simulink model "Boost_Converter"  (R2022b)
settings: Solver=VariableStepAuto  StartTime=0.0  StopTime=0.1  RelTol=1e-3
libraries: spsSeriesRLCBranchLib x3, spsMultimeterLib x2, spsDiodeLib x1, spsMeanLib x1, spsMosfetLib x1, spsPWMGeneratorDCDCLib x1, spsDCVoltageSourceLib x1, sps_lib x1
settings Model: Creator=Biplov Jha  LastModifiedBy=Biplov Jha

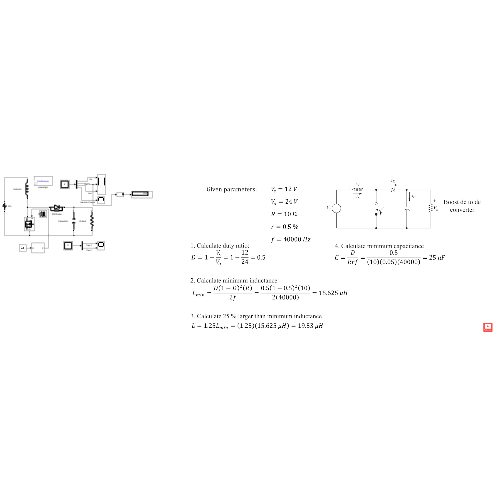
[thumbnail: Simulink's stored preview of the top-level diagram]
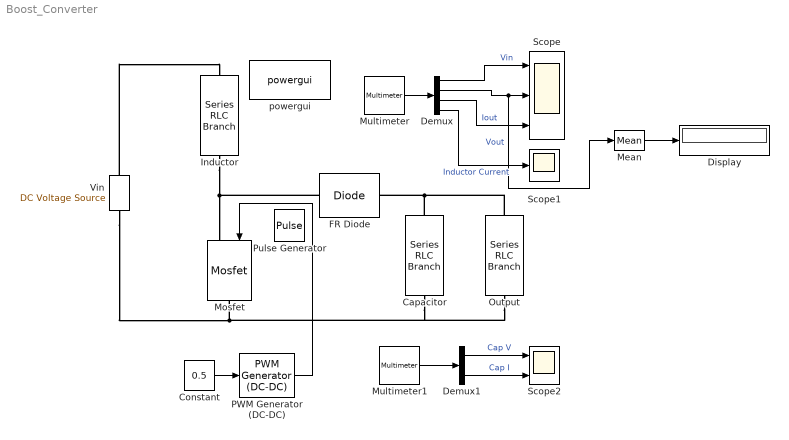
== system Boost_Converter ==
  Capacitor : spsSeriesRLCBranchLib/Series RLC Branch  LConnTagsString=__new0  RConnTagsString=__new0  BranchType=C  Resistance=1  Inductance=1e-3  SetiL0=off  InitialCurrent=0  Capacitance=25e-6  Setx0=off  InitialVoltage=0  Measurements=Branch voltage and current
  Constant : Constant  Value=0.5
  Demux : Demux
  Demux1 : Demux  Outputs=2
  Display : Display
  FR Diode : spsDiodeLib/Diode  Ron=0.001  Lon=0  Vf=0.8  IC=0  UseSnubber=0  Rs=500  Cs=250e-9  Measurements=off
  Inductor : spsSeriesRLCBranchLib/Series RLC Branch  LConnTagsString=__new0  RConnTagsString=__new0  BranchType=L  Resistance=1  Inductance=20e-6  SetiL0=off  InitialCurrent=0  Capacitance=1e-6  Setx0=off  InitialVoltage=0  Measurements=Branch current
  Mean : spsMeanLib/Mean  Freq=60  Vinit=0  Ts=0
  Mosfet : spsMosfetLib/Mosfet  Ron=0.1  Lon=0  Rd=0.01  Vfd=0  IC=0  Rs=1e5  Cs=inf  Measurements=off
  Multimeter : spsMultimeterLib/Multimeter  L=6  sel=[3 2 6 5]  yselected={}  Gain=[1 1 1 1]  OutputType=Complex  PlotAtSimulationStop=off  PhasorSimulation=off
  Multimeter1 : spsMultimeterLib/Multimeter  L=6  sel=[1 4]  yselected={}  Gain=[1 1]  OutputType=Complex  PlotAtSimulationStop=off  PhasorSimulation=off
  Output : spsSeriesRLCBranchLib/Series RLC Branch  LConnTagsString=__new0  RConnTagsString=__new0  BranchType=R  Resistance=10  Inductance=1e-3  SetiL0=off  InitialCurrent=0  Capacitance=1e-6  Setx0=off  InitialVoltage=0  Measurements=Branch voltage and current
  PWM Generator (DC-DC) : spsPWMGeneratorDCDCLib/PWM Generator (DC-DC)  Fsw=40000  Ts=0
  Pulse Generator : DiscretePulseGenerator  PulseType=Time based  Period=1/(40e3)  PulseWidth=50
  Scope : Scope  NumInputPorts=3
  Scope1 : Scope
  Scope2 : Scope  NumInputPorts=2
  Vin : spsDCVoltageSourceLib/DC Voltage Source  Amplitude=12  Measurements=Voltage
  powergui : sps_lib/powergui  Priority=1  SimulationMode=Continuous  SampleTime=50e-6  frequency=60  Iterations=50  frequencyindice=0  Pbase=100e6  ErrMax=1e-4  UnitsV=kV  UnitsW=MW  buscounter=0  FunctionMessages=off  echomessages=off  EnableUseOfTLC=off  CurrentSourceSwitches=off  DisableSnubberDevices=off  DisableRonSwitches=off  DisableVfSwitches=off  DisplayEquations=off  AutomaticDiscreteSolvers=off  SolverType=Tustin/Backward Euler (TBE)  Interpol=off  ExternalGateDelay=off  methode=off  Ts=100  x0status=blocks  SPID=on  SwTol=0  HookPort=off  NonlinearTolerance=1e-4  nMaxIteration=100  ContinueOnMaxIteration=off  RestoreLinks=warning  ResistiveCurrentMeasurement=off  Frange=[0:2:500]  Ylog=off  Xlog=on  ShowGrid=off  save=off  variable=ZData  structure=0  ZoomFFT=off  StartTime=0.0  cycles=1  DisplayStyle=1  fundamental=60  FreqAxis=off  MaxFrequency=1000  frequencyindicesteady=1  RmsSteady=1  display=off
  wires:
  Multimeter/1 -> Demux/1
  Demux/2 -> Mean/1, Scope/2  "Vout"
  Demux/1 -> Scope/1  "Vin"
  Demux/3 -> Scope/3  "Iout"
  Demux/4 -> Scope1/1  "Inductor Current"
  Mean/1 -> Display/1
  Multimeter1/1 -> Demux1/1
  Demux1/1 -> Scope2/1  "Cap V"
  Demux1/2 -> Scope2/2  "Cap I"
  Constant/1 -> PWM Generator (DC-DC)/1
  PWM Generator (DC-DC)/1 -> Mosfet/1
  connections:
  Vin/RConn1 -- Inductor/LConn1
  Vin/LConn1 -- Capacitor/RConn1 -- Output/RConn1 -- Mosfet/RConn1
  Inductor/RConn1 -- FR Diode/LConn1 -- Mosfet/LConn1
  Capacitor/LConn1 -- FR Diode/RConn1 -- Output/LConn1
